simulink model "ImmersionModelCombined"  (R2022b)
settings: Solver=FixedStepAuto  StartTime=0.0  StopTime=1200  FixedStep=0.1  RelTol=1e-3  EnableMultiTasking=on
undefined symbols (not defined in the file or in its folder): sigbuilder_block
libraries: SignalEditorBlockLib x6
settings Model: SimulationMode=rapid-accelerator  PacingRate=4  Creator=djstrauss  LastModifiedBy=strau
settings SolverCC: AlgebraicLoopSolver=TrustRegion
settings DataIOCC: LimitDataPoints=on  SaveFinalState=on  SaveFormat=Array  SaveState=on  InspectSignalLogs=on  LoggingToFile=on
settings OptimizationCC: LifeSpan=inf
settings DebuggingCC: UnconnectedInputMsg=warning  UnconnectedOutputMsg=warning  UnconnectedLineMsg=warning  SFUnexpectedBacktrackingDiag=warning  SFNoUnconditionalDefaultTransitionDiag=warning  SFExecutionAtInitializationDiag=none  SFMachineParentedDataDiag=warning  ArithmeticOperatorsInVariantConditions=warning
settings HardwareCC: ProdBitPerPointer=32  ProdBitPerSizeT=32  ProdBitPerPtrDiffT=32  ProdLargestAtomicFloat=None  ProdIntDivRoundTo=Undefined  ProdEndianess=Unspecified  ProdWordSize=32  ProdHWDeviceType=32-bit Generic
settings ModelReferenceCC: EnableRefExpFcnMdlSchedulingChecks=on  PropagateSignalLabelsOutOfModel=off
settings SFSimCC: SimUseLocalCustomCode=off  CustomCodeUndefinedFunction=UseInterfaceOnly
settings RTWCC: RTWUseLocalCustomCode=off  DLArmComputeVersion=19.05
settings CodeAppCC: StateflowObjectComments=on
settings GRTTargetCC: TargetLangStandard=C89/C90 (ANSI)
settings ConfigComp: CovMetricSettings=dw  CovSaveCumulativeToWorkspaceVar=on  CovSaveSingleToWorkspaceVar=on  CovExternalEMLEnable=off

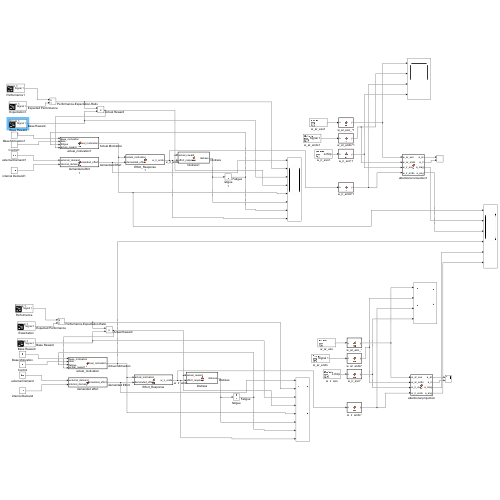
[thumbnail: Simulink's stored preview of the top-level diagram]
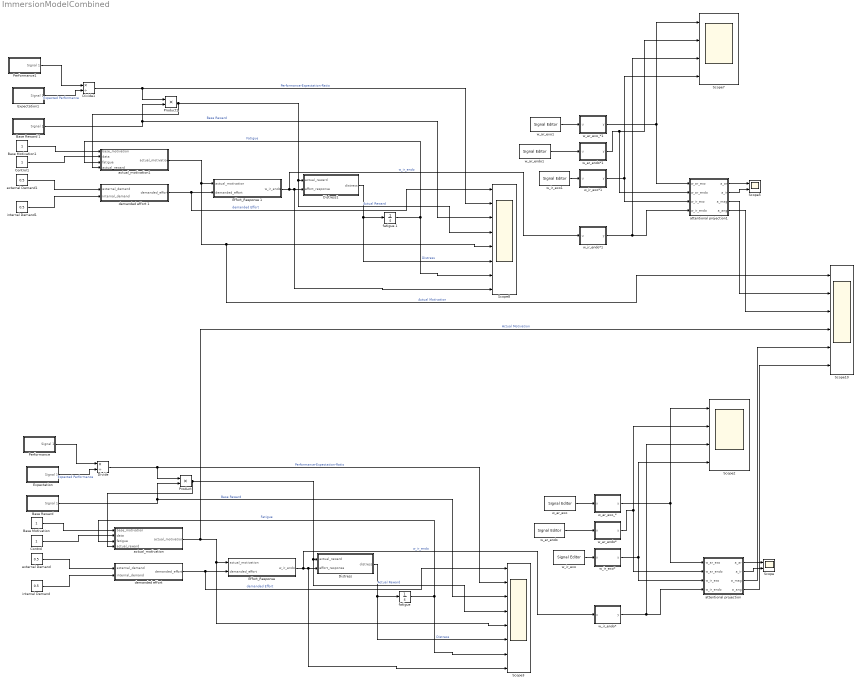
== system ImmersionModelCombined ==
  " Base Reward " : Subsystem  Tag=STV Subsys  LoadFcn=sigbuilder_block('load',[506.25 147.75 550.5 359.25 ]);  StartFcn=sigbuilder_block('start');  StopFcn=sigbuilder_block('stop');  ClipboardFcn=sigbuilder_block('clipboard');  mask(Sigbuilder block){tuvar=[0:10]}
      mask help: Simulink:masks:SigbuilderBlock_MD
      mask init:
      | if ~strcmp(get_param(bdroot(gcbh),'SimulationStatus'),'stopped') tuvar = sigbuilder_block('maskInit'); end
      settings: CopyFcn=sigbuilder_block('copy');  DeleteFcn=sigbuilder_block('delete');  ModelCloseFcn=sigbuilder_block('modelClose');  PreSaveFcn=sigbuilder_block('preSave');  PauseFcn=sigbuilder_block('pause');  ContinueFcn=sigbuilder_block('continue');  NameChangeFcn=sigbuilder_block('namechange');  OpenFcn=sigbuilder_block('open',[506.25 147.75 550.5 359.25 ]);  CloseFcn=sigbuilder_block('close');
      mask Display: plot(0, 0, 100, 100,[2, 2, 32, 32, 2], [68, 8, 8, 68, 68],[32, 2], [38, 38], [32, 19, 2],[53, 60, 44], [32, 17, 17, 2],[16, 16, 31, 31]);txt = getActiveGroup(gcbh);text(2, 100, txt,'verticalAlignment', 'top');
  " Base Reward 1" : Subsystem  Tag=STV Subsys  LoadFcn=sigbuilder_block('load',[506.25 147.75 550.5 357.75 ]);  StartFcn=sigbuilder_block('start');  StopFcn=sigbuilder_block('stop');  ClipboardFcn=sigbuilder_block('clipboard');  mask(Sigbuilder block){tuvar=[0:10]}
      mask help: Simulink:masks:SigbuilderBlock_MD
      mask init:
      | if ~strcmp(get_param(bdroot(gcbh),'SimulationStatus'),'stopped') tuvar = sigbuilder_block('maskInit'); end
      settings: CopyFcn=sigbuilder_block('copy');  DeleteFcn=sigbuilder_block('delete');  ModelCloseFcn=sigbuilder_block('modelClose');  PreSaveFcn=sigbuilder_block('preSave');  PauseFcn=sigbuilder_block('pause');  ContinueFcn=sigbuilder_block('continue');  NameChangeFcn=sigbuilder_block('namechange');  OpenFcn=sigbuilder_block('open',[506.25 147.75 550.5 357.75 ]);  CloseFcn=sigbuilder_block('close');
      mask Display: plot(0, 0, 100, 100,[2, 2, 32, 32, 2], [68, 8, 8, 68, 68],[32, 2], [38, 38], [32, 19, 2],[53, 60, 44], [32, 17, 17, 2],[16, 16, 31, 31]);txt = getActiveGroup(gcbh);text(2, 100, txt,'verticalAlignment', 'top');
  Base Motivation : Constant
  Base Motivation1 : Constant
  Control : Constant
  Control1 : Constant
  Distress : MATLAB Function  TreatAsAtomicUnit=on
  Distress1 : MATLAB Function  TreatAsAtomicUnit=on
  Divide : Product  Inputs=*/
  Divide1 : Product  Inputs=*/
  "Effort_Response " : MATLAB Function  TreatAsAtomicUnit=on
  Effort_Response 1 : MATLAB Function  TreatAsAtomicUnit=on
  Expectation : Subsystem  Tag=STV Subsys  LoadFcn=sigbuilder_block('load');  StartFcn=sigbuilder_block('start');  StopFcn=sigbuilder_block('stop');  ClipboardFcn=sigbuilder_block('clipboard');  mask(Sigbuilder block){tuvar=[0:10]}
      mask help: Simulink:masks:SigbuilderBlock_MD
      mask init:
      | if ~strcmp(get_param(bdroot(gcbh),'SimulationStatus'),'stopped') tuvar = sigbuilder_block('maskInit'); end
      settings: CopyFcn=sigbuilder_block('copy');  DeleteFcn=sigbuilder_block('delete');  ModelCloseFcn=sigbuilder_block('modelClose');  PreSaveFcn=sigbuilder_block('preSave');  PauseFcn=sigbuilder_block('pause');  ContinueFcn=sigbuilder_block('continue');  NameChangeFcn=sigbuilder_block('namechange');  OpenFcn=sigbuilder_block('open',[0 36 1125 661.5 ]);  CloseFcn=sigbuilder_block('close');
      mask Display: plot(0, 0, 100, 100,[2, 2, 32, 32, 2], [68, 8, 8, 68, 68],[32, 2], [38, 38], [32, 19, 2],[53, 60, 44], [32, 17, 17, 2],[16, 16, 31, 31]);txt = getActiveGroup(gcbh);text(2, 100, txt,'verticalAlignment', 'top');
  Expectation1 : Subsystem  Tag=STV Subsys  LoadFcn=sigbuilder_block('load');  StartFcn=sigbuilder_block('start');  StopFcn=sigbuilder_block('stop');  ClipboardFcn=sigbuilder_block('clipboard');  mask(Sigbuilder block){tuvar=[0:10]}
      mask help: Simulink:masks:SigbuilderBlock_MD
      mask init:
      | if ~strcmp(get_param(bdroot(gcbh),'SimulationStatus'),'stopped') tuvar = sigbuilder_block('maskInit'); end
      settings: CopyFcn=sigbuilder_block('copy');  DeleteFcn=sigbuilder_block('delete');  ModelCloseFcn=sigbuilder_block('modelClose');  PreSaveFcn=sigbuilder_block('preSave');  PauseFcn=sigbuilder_block('pause');  ContinueFcn=sigbuilder_block('continue');  NameChangeFcn=sigbuilder_block('namechange');  OpenFcn=sigbuilder_block('open',[6 30 1012.5 447.75 ]);  CloseFcn=sigbuilder_block('close');
      mask Display: plot(0, 0, 100, 100,[2, 2, 32, 32, 2], [68, 8, 8, 68, 68],[32, 2], [38, 38], [32, 19, 2],[53, 60, 44], [32, 17, 17, 2],[16, 16, 31, 31]);txt = getActiveGroup(gcbh);text(2, 100, txt,'verticalAlignment', 'top');
  Performance : Subsystem  Tag=STV Subsys  LoadFcn=sigbuilder_block('load');  StartFcn=sigbuilder_block('start');  StopFcn=sigbuilder_block('stop');  ClipboardFcn=sigbuilder_block('clipboard');  mask(Sigbuilder block){tuvar=[0:10]}
      mask help: Simulink:masks:SigbuilderBlock_MD
      mask init:
      | if ~strcmp(get_param(bdroot(gcbh),'SimulationStatus'),'stopped') tuvar = sigbuilder_block('maskInit'); end
      settings: CopyFcn=sigbuilder_block('copy');  DeleteFcn=sigbuilder_block('delete');  ModelCloseFcn=sigbuilder_block('modelClose');  PreSaveFcn=sigbuilder_block('preSave');  PauseFcn=sigbuilder_block('pause');  ContinueFcn=sigbuilder_block('continue');  NameChangeFcn=sigbuilder_block('namechange');  OpenFcn=sigbuilder_block('open',[6 33 1012.5 444 ]);  CloseFcn=sigbuilder_block('close');
      mask Display: plot(0, 0, 100, 100,[2, 2, 32, 32, 2], [68, 8, 8, 68, 68],[32, 2], [38, 38], [32, 19, 2],[53, 60, 44], [32, 17, 17, 2],[16, 16, 31, 31]);txt = getActiveGroup(gcbh);text(2, 100, txt,'verticalAlignment', 'top');
  Performance1 : Subsystem  Tag=STV Subsys  LoadFcn=sigbuilder_block('load');  StartFcn=sigbuilder_block('start');  StopFcn=sigbuilder_block('stop');  ClipboardFcn=sigbuilder_block('clipboard');  mask(Sigbuilder block){tuvar=[0:10]}
      mask help: Simulink:masks:SigbuilderBlock_MD
      mask init:
      | if ~strcmp(get_param(bdroot(gcbh),'SimulationStatus'),'stopped') tuvar = sigbuilder_block('maskInit'); end
      settings: CopyFcn=sigbuilder_block('copy');  DeleteFcn=sigbuilder_block('delete');  ModelCloseFcn=sigbuilder_block('modelClose');  PreSaveFcn=sigbuilder_block('preSave');  PauseFcn=sigbuilder_block('pause');  ContinueFcn=sigbuilder_block('continue');  NameChangeFcn=sigbuilder_block('namechange');  OpenFcn=sigbuilder_block('open',[6 33 1012.5 444 ]);  CloseFcn=sigbuilder_block('close');
      mask Display: plot(0, 0, 100, 100,[2, 2, 32, 32, 2], [68, 8, 8, 68, 68],[32, 2], [38, 38], [32, 19, 2],[53, 60, 44], [32, 17, 17, 2],[16, 16, 31, 31]);txt = getActiveGroup(gcbh);text(2, 100, txt,'verticalAlignment', 'top');
  Product : Product
  Product1 : Product
  Scope : Scope  NumInputPorts=2
  Scope10 : Scope  NumInputPorts=6
  Scope2 : Scope  NumInputPorts=4
  Scope3 : Scope  NumInputPorts=8
  Scope5 : Scope  NumInputPorts=2
  Scope7 : Scope  NumInputPorts=4
  Scope8 : Scope  NumInputPorts=8
  actual_motivation : MATLAB Function  TreatAsAtomicUnit=on
  actual_motivation1 : MATLAB Function  TreatAsAtomicUnit=on
  attentional projection : MATLAB Function  TreatAsAtomicUnit=on
  attentional projection1 : MATLAB Function  TreatAsAtomicUnit=on
  "demanded effort " : MATLAB Function  TreatAsAtomicUnit=on
  demanded effort 1 : MATLAB Function  TreatAsAtomicUnit=on
  external Demand : Constant  Value=0.5
  external Demand1 : Constant  Value=0.5
  "fatigue " : Integrator
  fatigue 1 : Integrator
  internal Demand : Constant  Value=0.5
  internal Demand1 : Constant  Value=0.5
  w_ar_endo : SignalEditorBlockLib/Signal Editor  FileName=sinewave.mat  ActiveScenario=Scenario  ActiveSignal=Signal 1  IsBus=off  OutputBusObjectStr=Bus: BusObject  SampleTime=0  Interpolate=off  ZeroCross=off  OutputAfterFinalValue=Setting to zero  Unit=inherit  PreserveSignalName=on
  w_ar_endo* : MATLAB Function  TreatAsAtomicUnit=on
  w_ar_endo*1 : MATLAB Function  TreatAsAtomicUnit=on
  w_ar_endo1 : SignalEditorBlockLib/Signal Editor  FileName=sinewave.mat  ActiveScenario=Scenario  ActiveSignal=Signal 1  IsBus=off  OutputBusObjectStr=Bus: BusObject  SampleTime=0  Interpolate=off  ZeroCross=off  OutputAfterFinalValue=Setting to zero  Unit=inherit  PreserveSignalName=on
  w_ar_exo : SignalEditorBlockLib/Signal Editor  FileName=C:\SNNU\Projects\Immersion\GImpulse.mat  ActiveScenario=Scenario  ActiveSignal=.  IsBus=off  OutputBusObjectStr=Bus: BusObject  SampleTime=0  Interpolate=off  ZeroCross=off  OutputAfterFinalValue=Setting to zero  Unit=inherit  PreserveSignalName=on
  w_ar_exo1 : SignalEditorBlockLib/Signal Editor  FileName=C:\SNNU\Projects\Immersion\GImpulse.mat  ActiveScenario=Scenario  ActiveSignal=.  IsBus=off  OutputBusObjectStr=Bus: BusObject  SampleTime=0  Interpolate=off  ZeroCross=off  OutputAfterFinalValue=Setting to zero  Unit=inherit  PreserveSignalName=on
  w_ar_exo_* : MATLAB Function  TreatAsAtomicUnit=on
  w_ar_exo_*1 : MATLAB Function  TreatAsAtomicUnit=on
  w_ir_endo* : MATLAB Function  TreatAsAtomicUnit=on
  w_ir_endo*1 : MATLAB Function  TreatAsAtomicUnit=on
  w_ir_exo : SignalEditorBlockLib/Signal Editor  FileName=C:\SNNU\Projects\Immersion\LChirpsig.mat  ActiveScenario=Scenario  ActiveSignal=Lchirp  IsBus=off  OutputBusObjectStr=Bus: BusObject  SampleTime=0  Interpolate=off  ZeroCross=off  OutputAfterFinalValue=Setting to zero  Unit=inherit  PreserveSignalName=on
  w_ir_exo* : MATLAB Function  TreatAsAtomicUnit=on
  w_ir_exo*1 : MATLAB Function  TreatAsAtomicUnit=on
  w_ir_exo1 : SignalEditorBlockLib/Signal Editor  FileName=C:\SNNU\Projects\Immersion\LChirpsig.mat  ActiveScenario=Scenario  ActiveSignal=Lchirp  IsBus=off  OutputBusObjectStr=Bus: BusObject  SampleTime=0  Interpolate=off  ZeroCross=off  OutputAfterFinalValue=Setting to zero  Unit=inherit  PreserveSignalName=on
  wires:
  attentional projection/1(a_ar) -> Scope/1
  attentional projection/2(a_ir) -> Scope/2
  Expectation/1(Signal 1) -> Divide/2  "Expected Performance"
  Divide/1 -> Scope3/2, Product/1  "Performance-Expectation-Ratio"
  "Effort_Response "/1(w_ir_endo) -> w_ir_endo*/1(u), Scope3/8, Distress/2(effort_response)  "w_ir_endo"
  internal Demand/1 -> "demanded effort "/2(internal_demand)
  Distress/1(distress) -> Scope3/6, "fatigue "/1  "Distress"
  actual_motivation/1(actual_motivation) -> Scope10/4, Scope3/5, "Effort_Response "/1(actual_motivation)  "Actual Motivation"
  Product/1 -> actual_motivation/4(actual_reward), Scope3/4, Distress/1(actual_reward)  "Actual Reward"
  Control/1 -> actual_motivation/2(data)
  " Base Reward "/1(Signal 1) -> Product/2, Scope3/3  "Base Reward"
  Base Motivation/1 -> actual_motivation/1(base_motivation)
  external Demand/1 -> "demanded effort "/1(external_demand)
  "demanded effort "/1(demanded_effort) -> Scope3/1, "Effort_Response "/2(demanded_effort)  "demanded Effort"
  "fatigue "/1 -> Scope3/7, actual_motivation/3(fatigue)  "Fatigue"
  w_ar_endo*/1(y) -> Scope2/2, attentional projection/2(w_ar_endo)
  w_ar_endo/1 -> w_ar_endo*/1(u)
  w_ar_exo/1 -> w_ar_exo_*/1(u)
  w_ar_exo_*/1(y) -> Scope2/1, attentional projection/1(w_ar_exo)
  w_ir_exo/1 -> w_ir_exo*/1(u)
  w_ir_exo*/1(y) -> Scope2/4, attentional projection/3(w_ir_exo)
  w_ir_endo*/1(y) -> Scope2/3, attentional projection/4(w_ir_endo)
  Performance/1(Signal 1) -> Divide/1
  " Base Reward 1"/1(Signal 1) -> Product1/2, Scope8/3  "Base Reward"
  Product1/1 -> actual_motivation1/4(actual_reward), Scope8/4, Distress1/1(actual_reward)  "Actual Reward"
  internal Demand1/1 -> demanded effort 1/2(internal_demand)
  Control1/1 -> actual_motivation1/2(data)
  attentional projection1/1(a_ar) -> Scope5/1
  Distress1/1(distress) -> Scope8/6, fatigue 1/1  "Distress"
  Performance1/1(Signal 1) -> Divide1/1
  w_ar_exo1/1 -> w_ar_exo_*1/1(u)
  w_ar_exo_*1/1(y) -> Scope7/1, attentional projection1/1(w_ar_exo)
  w_ir_endo*1/1(y) -> Scope7/3, attentional projection1/4(w_ir_endo)
  w_ir_exo*1/1(y) -> Scope7/4, attentional projection1/3(w_ir_exo)
  Divide1/1 -> Scope8/2, Product1/1  "Performance-Expectation-Ratio"
  external Demand1/1 -> demanded effort 1/1(external_demand)
  w_ir_exo1/1 -> w_ir_exo*1/1(u)
  Base Motivation1/1 -> actual_motivation1/1(base_motivation)
  Expectation1/1(Signal 1) -> Divide1/2  "Expected Performance"
  attentional projection1/2(a_ir) -> Scope5/2
  Effort_Response 1/1(w_ir_endo) -> w_ir_endo*1/1(u), Scope8/8, Distress1/2(effort_response)  "w_ir_endo"
  demanded effort 1/1(demanded_effort) -> Scope8/1, Effort_Response 1/2(demanded_effort)  "demanded Effort"
  w_ar_endo1/1 -> w_ar_endo*1/1(u)
  actual_motivation1/1(actual_motivation) -> Scope10/1, Scope8/5, Effort_Response 1/1(actual_motivation)  "Actual Motivation"
  w_ar_endo*1/1(y) -> Scope7/2, attentional projection1/2(w_ar_endo)
  fatigue 1/1 -> Scope8/7, actual_motivation1/3(fatigue)  "Fatigue"
  attentional projection1/4(a_ang) -> Scope10/3
  attentional projection1/3(a_mag) -> Scope10/2
  attentional projection/4(a_ang) -> Scope10/6
  attentional projection/3(a_mag) -> Scope10/5

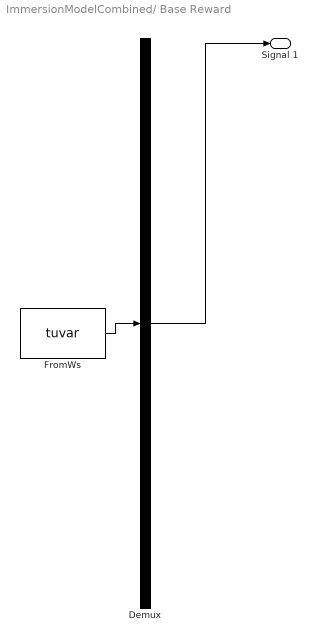
== system ImmersionModelCombined/ Base Reward  ==
  Demux : Demux  Tag=STV Demux  Outputs=1
      settings: DisplayOption=none
  FromWs : FromWorkspace  Tag=STV FromWs  VariableName=tuvar
      SigBuilderData=|
      | common.afterFinalStr = 'Extrapolate'
      | common.sampleTime = 0
      | dataSet.timeRange = [0 1200]
      | dataSet.name = 'Group 1'
      | sbobj.Groups.Name = 'Group 1'
      | sbobj.Groups.Signals.Name = 'Signal 1'
      | sbobj.Groups.Signals.XData = [0 200 400 498 600 704 800 1010 1200]
      | sbobj.Groups.Signals.YData = [0.51 0.585 0.62 0.575 0.39 0.195 0.1 0.02 -0.005]
      | sbobj.Groups.TimeRange = [0 1200]
  Signal 1 : Outport  Tag=STV Outport
  wires:
  Demux/1 -> Signal 1/1
  FromWs/1 -> Demux/1

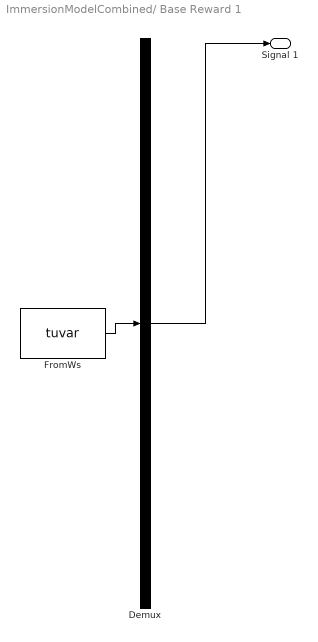
== system ImmersionModelCombined/ Base Reward 1 ==
  Demux : Demux  Tag=STV Demux  Outputs=1
      settings: DisplayOption=none
  FromWs : FromWorkspace  Tag=STV FromWs  VariableName=tuvar
      SigBuilderData=|
      | common.afterFinalStr = 'Extrapolate'
      | common.sampleTime = 0
      | dataSet.timeRange = [0 1200]
      | dataSet.name = 'Group 1'
      | sbobj.Groups.Name = 'Group 1'
      | sbobj.Groups.Signals.Name = 'Signal 1'
      | sbobj.Groups.Signals.XData = [0 200 400 498 600 704 800 1010 1200]
      | sbobj.Groups.Signals.YData = [0.245 0.515 0.67 0.75 0.88 0.945 0.955 0.98 0.985]
      | sbobj.Groups.TimeRange = [0 1200]
  Signal 1 : Outport  Tag=STV Outport
  wires:
  Demux/1 -> Signal 1/1
  FromWs/1 -> Demux/1

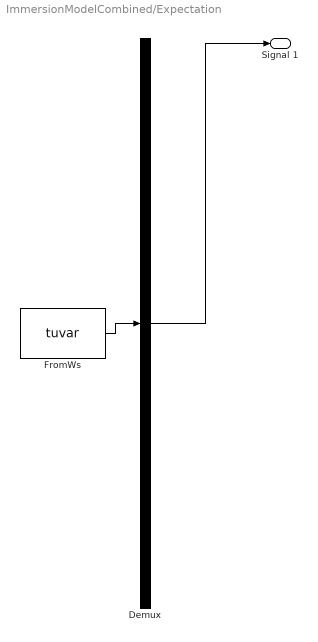
== system ImmersionModelCombined/Expectation ==
  Demux : Demux  Tag=STV Demux  Outputs=1
      settings: DisplayOption=none
  FromWs : FromWorkspace  Tag=STV FromWs  VariableName=tuvar
      SigBuilderData=|
      | common.afterFinalStr = 'Extrapolate'
      | common.sampleTime = 0
      | dataSet.timeRange = [0 1200]
      | dataSet.name = 'Group 1'
      | sbobj.Groups.Name = 'Group 1'
      | sbobj.Groups.Signals.Name = 'Signal 1'
      | sbobj.Groups.Signals.XData = [0 1200]
      | sbobj.Groups.Signals.YData = [0.5 0.5]
      | sbobj.Groups.TimeRange = [0 1200]
  Signal 1 : Outport  Tag=STV Outport
  wires:
  Demux/1 -> Signal 1/1
  FromWs/1 -> Demux/1

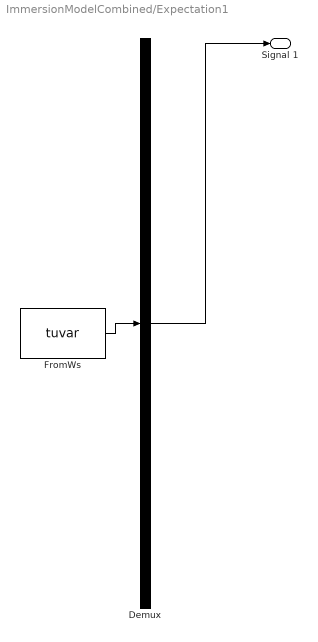
== system ImmersionModelCombined/Expectation1 ==
  Demux : Demux  Tag=STV Demux  Outputs=1
      settings: DisplayOption=none
  FromWs : FromWorkspace  Tag=STV FromWs  VariableName=tuvar
      SigBuilderData=|
      | common.afterFinalStr = 'Extrapolate'
      | common.sampleTime = 0
      | dataSet.timeRange = [0 1200]
      | dataSet.name = 'Group 1'
      | sbobj.Groups.Name = 'Group 1'
      | sbobj.Groups.Signals.Name = 'Signal 1'
      | sbobj.Groups.Signals.XData = [0 1200]
      | sbobj.Groups.Signals.YData = [0.5 0.5]
      | sbobj.Groups.TimeRange = [0 1200]
  Signal 1 : Outport  Tag=STV Outport
  wires:
  Demux/1 -> Signal 1/1
  FromWs/1 -> Demux/1

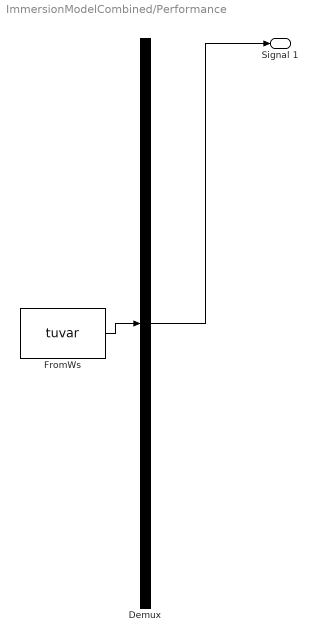
== system ImmersionModelCombined/Performance ==
  Demux : Demux  Tag=STV Demux  Outputs=1
      settings: DisplayOption=none
  FromWs : FromWorkspace  Tag=STV FromWs  VariableName=tuvar
      SigBuilderData=|
      | common.afterFinalStr = 'Extrapolate'
      | common.sampleTime = 0
      | dataSet.timeRange = [0 1200]
      | dataSet.name = 'Group 1'
      | sbobj.Groups.Name = 'Group 1'
      | sbobj.Groups.Signals.Name = 'Signal 1'
      | sbobj.Groups.Signals.XData = [0 600 1200]
      | sbobj.Groups.Signals.YData = [0.5 0.5 0.5]
      | sbobj.Groups.TimeRange = [0 1200]
  Signal 1 : Outport  Tag=STV Outport
  wires:
  Demux/1 -> Signal 1/1
  FromWs/1 -> Demux/1

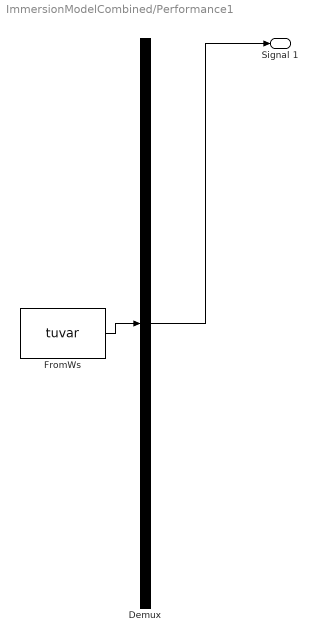
== system ImmersionModelCombined/Performance1 ==
  Demux : Demux  Tag=STV Demux  Outputs=1
      settings: DisplayOption=none
  FromWs : FromWorkspace  Tag=STV FromWs  VariableName=tuvar
      SigBuilderData=|
      | common.afterFinalStr = 'Extrapolate'
      | common.sampleTime = 0
      | dataSet.timeRange = [0 1200]
      | dataSet.name = 'Group 1'
      | sbobj.Groups.Name = 'Group 1'
      | sbobj.Groups.Signals.Name = 'Signal 1'
      | sbobj.Groups.Signals.XData = [0 600 1200]
      | sbobj.Groups.Signals.YData = [0.5 0.5 0.5]
      | sbobj.Groups.TimeRange = [0 1200]
  Signal 1 : Outport  Tag=STV Outport
  wires:
  Demux/1 -> Signal 1/1
  FromWs/1 -> Demux/1

== matlab function ImmersionModelCombined/actual_motivation1 ==
  data: base_motivation input; data input; fatigue input; actual_motivation output; actual_reward input
function actual_motivation = fcn(base_motivation,  data, fatigue, actual_reward)%control,

alpha=1.0;beta=0.05; 
actual_motivation=(base_motivation+exp(-((fatigue.^2)*beta))*data*actual_reward)-alpha;

== matlab function ImmersionModelCombined/attentional projection1 ==
  data: a_ar output; w_ar_exo input; w_ar_endo input; w_ir_exo input; w_ir_endo input; a_ir output; a_mag output; a_ang output
function [a_ar,a_ir,a_mag,a_ang] = fcn(w_ar_exo,w_ar_endo,w_ir_exo,w_ir_endo)

% a_ar=tanh(3.5*(omega_ar_exo+omega_ar_endo));
% a_ir=tanh(3.5*(omega_ir_exo+omega_ir_endo));
%alpha=1.0; beta=3.25; rho=0.0;

% 
% a_ar=w_ar_exo+(alpha-max(w_ar_exo-rho,0))*w_ar_endo;
% a_ir=w_ir_exo+(alpha-max(w_ir_exo-rho,0))*w_ir_endo;

%a_ar=alpha.*tanh(beta.*(w_ar_exo+w_ar_endo));
%a_ir=alpha.*tanh(beta.*(w_ir_exo+w_ir_endo));

a_ar=w_ar_exo+w_ar_endo;
a_ir=w_ir_exo+w_ir_endo;

% 
%  nf=a_ar+a_ir;
% % 
%      a_ar=a_ar/nf;
%      a_ir=a_ir/nf;
    
a_mag=sqrt(a_ar.^2+a_ir.^2);
%a_mag=alpha.*tanh(beta.*a_mag);

a_ang=atand(a_ir./a_ar);

== matlab function ImmersionModelCombined/demanded effort 1 ==
  data: external_demand input; internal_demand input; demanded_effort output
function demanded_effort = fcn(external_demand, internal_demand)

 demanded_effort = sqrt(external_demand^2 + 2*internal_demand^2);
% demanded_effort = external_demand + internal_demand;

== matlab function ImmersionModelCombined/w_ar_endo*1 ==
  data: u input; y output
function y = fcn(u)

%alpha=1; beta=3.25;
%y = alpha.*(tanh(u.*beta));

alpha=0.42; beta=9; gamma=5;
y=(alpha)./(1+ exp(-((u)*beta)+gamma));

== matlab function ImmersionModelCombined/actual_motivation ==
  data: base_motivation input; data input; fatigue input; actual_motivation output; actual_reward input
function actual_motivation = fcn(base_motivation,  data, fatigue, actual_reward)%control,

alpha=1.0;beta=0.05; 
actual_motivation=(base_motivation+exp(-((fatigue.^2)*beta))*data*actual_reward)-alpha;

== matlab function ImmersionModelCombined/w_ar_exo_*1 ==
  data: u input; y output
function y = fcn(u)

%alpha=1; beta=3.25;
%y = alpha.*(tanh(u.*beta));

alpha=0.58; beta=7; gamma=5;
y=(alpha)./(1+ exp(-((u)*beta)+gamma));

== matlab function ImmersionModelCombined/w_ir_endo*1 ==
  data: u input; y output
function y = fcn(u)

%alpha=1; beta=3.25;
%y = alpha.*(tanh(u.*beta));
u=2.*u;
alpha=0.42; beta=9; gamma=5;
y=(alpha)./(1+ exp(-((u)*beta)+gamma));

== matlab function ImmersionModelCombined/w_ir_exo*1 ==
  data: u input; y output
function y = fcn(u)

%alpha=1; beta=3.25;
%y = alpha.*(tanh(u.*beta));

alpha=0.58; beta=7; gamma=5;
y=(alpha)./(1+ exp(-((u)*beta)+gamma));

== matlab function ImmersionModelCombined/attentional projection ==
  data: a_ar output; w_ar_exo input; w_ar_endo input; w_ir_exo input; w_ir_endo input; a_ir output; a_mag output; a_ang output
function [a_ar,a_ir,a_mag,a_ang] = fcn(w_ar_exo,w_ar_endo,w_ir_exo,w_ir_endo)

% a_ar=tanh(3.5*(omega_ar_exo+omega_ar_endo));
% a_ir=tanh(3.5*(omega_ir_exo+omega_ir_endo));
%alpha=1.0; beta=3.25; rho=0.0;

% 
% a_ar=w_ar_exo+(alpha-max(w_ar_exo-rho,0))*w_ar_endo;
% a_ir=w_ir_exo+(alpha-max(w_ir_exo-rho,0))*w_ir_endo;

%a_ar=alpha.*tanh(beta.*(w_ar_exo+w_ar_endo));
%a_ir=alpha.*tanh(beta.*(w_ir_exo+w_ir_endo));

a_ar=w_ar_exo+w_ar_endo;
a_ir=w_ir_exo+w_ir_endo;

% 
%  nf=a_ar+a_ir;
% % 
%      a_ar=a_ar/nf;
%      a_ir=a_ir/nf;
    
a_mag=sqrt(a_ar.^2+a_ir.^2);
%a_mag=alpha.*tanh(beta.*a_mag);

a_ang=atand(a_ir./a_ar);

== matlab function ImmersionModelCombined/Effort_Response  ==
  data: actual_motivation input; w_ir_endo output; demanded_effort input
function w_ir_endo = fcn(actual_motivation, demanded_effort)

%if motivation == 1
    p=2.5;
    b=2.5;
% %else 
%     p=2.0;
%     b=2.0;
%end

unscaled_response=(((b^p)/gamma(1-demanded_effort))*demanded_effort.^(p-1)*exp(-b*(1-demanded_effort)));

w_ir_endo =max((actual_motivation)*unscaled_response,0);

== matlab function ImmersionModelCombined/Distress ==
  data: actual_reward input; effort_response input; distress output
function distress = fcn(actual_reward, effort_response)

if actual_reward < 0.01
    actual_reward=0.01;
end

arg=effort_response./actual_reward;

a=1; 
b=4;

distress = max((1./(1 + exp(-a*(arg-b))))-0.025 ,0);

== matlab function ImmersionModelCombined/demanded effort  ==
  data: external_demand input; internal_demand input; demanded_effort output
function demanded_effort = fcn(external_demand, internal_demand)

 demanded_effort = sqrt(external_demand^2 + 2*internal_demand^2);
% demanded_effort = external_demand + internal_demand;

== matlab function ImmersionModelCombined/w_ir_endo* ==
  data: u input; y output
function y = fcn(u)

%alpha=1; beta=3.25;
%y = alpha.*(tanh(u.*beta));
u=2.*u;
alpha=0.42; beta=9; gamma=5;
y=(alpha)./(1+ exp(-((u)*beta)+gamma));

== matlab function ImmersionModelCombined/w_ar_endo* ==
  data: u input; y output
function y = fcn(u)

%alpha=1; beta=3.25;
%y = alpha.*(tanh(u.*beta));

alpha=0.42; beta=9; gamma=5;
y=(alpha)./(1+ exp(-((u)*beta)+gamma));

== matlab function ImmersionModelCombined/w_ar_exo_* ==
  data: u input; y output
function y = fcn(u)

%alpha=1; beta=3.25;
%y = alpha.*(tanh(u.*beta));

alpha=0.58; beta=7; gamma=5;
y=(alpha)./(1+ exp(-((u)*beta)+gamma));

== matlab function ImmersionModelCombined/w_ir_exo* ==
  data: u input; y output
function y = fcn(u)

%alpha=1; beta=3.25;
%y = alpha.*(tanh(u.*beta));

alpha=0.58; beta=7; gamma=5;
y=(alpha)./(1+ exp(-((u)*beta)+gamma));

== matlab function ImmersionModelCombined/Distress1 ==
  data: actual_reward input; effort_response input; distress output
function distress = fcn(actual_reward, effort_response)

if actual_reward < 0.01
    actual_reward=0.01;
end

arg=effort_response./actual_reward;

a=1; 
b=4;

distress = max((1./(1 + exp(-a*(arg-b))))-0.025 ,0);

== matlab function ImmersionModelCombined/Effort_Response 1 ==
  data: actual_motivation input; w_ir_endo output; demanded_effort input
function w_ir_endo = fcn(actual_motivation, demanded_effort)

%if motivation == 1
    p=2.5;
    b=2.5;
% %else 
%     p=2.0;
%     b=2.0;
%end

unscaled_response=(((b^p)/gamma(1-demanded_effort))*demanded_effort.^(p-1)*exp(-b*(1-demanded_effort)));

w_ir_endo =max((actual_motivation)*unscaled_response,0);
